simulink library "qconvolution"  (R2015b)
settings: Solver=VariableStepAuto  StartTime=0.0  StopTime=10.0  RelTol=1e-3
values from neighbouring files (symbols this model uses):
  dt = 0.00005    (= 5e-05)    [param.m]
  freq = 5000    [param.m]
libraries: convolution x2
settings Model: Creator=mishuk  LastModifiedBy=mishuk

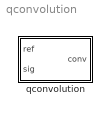
== system qconvolution ==
  qconvolution : Subsystem  mask{delay=0}
      mask prompts: delay "Refernce delay"
      mask help: Quadratic convolution of signal & reference delayed

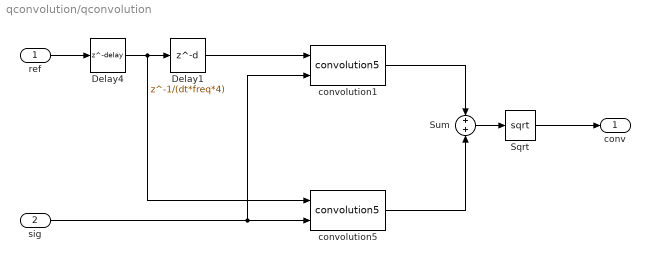
== system qconvolution/qconvolution ==
  ref : Inport
  sig : Inport  Port=2
  Delay1 : Delay  DelayLength=1/(dt*freq*4)
  Delay4 : Delay  DelayLength=delay
  Sqrt : Sqrt  SaturateOnIntegerOverflow=on
  Sum : Sum  Inputs=+|+
  convolution1 : convolution/convolution5  delay=delay
  convolution5 : convolution/convolution5  delay=delay
  conv : Outport
  wires:
  Delay1/1 -> convolution1/1
  sig/1 -> convolution1/2, convolution5/2
  convolution5/1 -> Sum/2
  convolution1/1 -> Sum/1
  Sqrt/1 -> conv/1
  Delay4/1 -> convolution5/1, Delay1/1
  Sum/1 -> Sqrt/1
  ref/1 -> Delay4/1
